simulink model "IEEE39_IBR_FrequencyControl_Fullversion_2020b"  (R2020b)
settings: Solver=VariableStepAuto  StartTime=0.0  StopTime=30  RelTol=1e-3
InitFcn:
  | IEEE39data_FrencyControl_full_Opensource;
undefined symbols (not defined in the file): alpha, c, eps_ps, eps_u, Fref, IBR_data, line, Sbase, t_start_disturbance, t_startcontrol, Vbase
libraries: powerlib x202, powerlib_meascontrol x81, powerlib_extras x27, pid_lib x14, simulink x4
(part 5 of 5)

== system IEEE39_IBR_FrequencyControl_Fullversion_2020b/G6_GFL/PV_PQ3/Subsystem2/Subsystem1 ==
  P_ref : Inport
  Q_ref : Inport  Port=2
  Ud : Inport  Port=3
  Divide5 : Product  Inputs=*/
  Divide6 : Product  Inputs=*/
  Gain1 : Gain  Gain=-2/3
  Gain2 : Gain  Gain=2/3
  Id_ref : Outport  VectorParamsAs1DForOutWhenUnconnected=off
  Iq_ref : Outport  Port=2  VectorParamsAs1DForOutWhenUnconnected=off
  wires:
  Q_ref/1 -> Divide6/1
  Divide6/1 -> Gain1/1
  P_ref/1 -> Divide5/1
  Gain1/1 -> Iq_ref/1
  Divide5/1 -> Gain2/1
  Gain2/1 -> Id_ref/1
  Ud/1 -> Divide6/2, Divide5/2

== system IEEE39_IBR_FrequencyControl_Fullversion_2020b/G6_GFL/PV_PQ3/Subsystem2/WL ==
  In1 : Inport
  freq : Inport  Port=2
  L : Inport  Port=3
  2pai : Constant  Value=2*pi
  Product : Product  Inputs=**
  Product1 : Product  Inputs=***
  Out1 : Outport  VectorParamsAs1DForOutWhenUnconnected=off
  wires:
  2pai/1 -> Product/2
  L/1 -> Product1/3
  freq/1 -> Product/1
  Product1/1 -> Out1/1
  Product/1 -> Product1/2
  In1/1 -> Product1/1

== system IEEE39_IBR_FrequencyControl_Fullversion_2020b/G6_GFL/PV_PQ3/Subsystem2/WL1 ==
  In1 : Inport
  freq : Inport  Port=2
  L : Inport  Port=3
  2pai : Constant  Value=2*pi
  Product : Product
  Product1 : Product  Inputs=3
  Out1 : Outport  VectorParamsAs1DForOutWhenUnconnected=off
  wires:
  2pai/1 -> Product/2
  L/1 -> Product1/3
  freq/1 -> Product/1
  Product1/1 -> Out1/1
  Product/1 -> Product1/2
  In1/1 -> Product1/1

== system IEEE39_IBR_FrequencyControl_Fullversion_2020b/GFM1/PV_PQ3/Freq_Droop/Subsystem1 ==
  w : Inport
  Add4 : Sum
  Clock : Clock
  Constant : Constant  Value=0
  Constant1 : Constant  Value=IBR_data(10,4)
  Constant2 : Constant  Value=IBR_data(10,5)
  Difference : simulink/Discrete/Difference  ICPrevInput=0.0  OutMin=[]  OutMax=[]  OutDataType=fixdt(1, 16)  OutScaling=2^-10  DoSatur=off
  Divide1 : Product  Inputs=**
  Divide3 : Product  Inputs=**
  Subsystem : Subsystem
  Switch : Switch  Criteria=u2 > Threshold  Threshold=t_startcontrol  ZeroCross=off
  Out1 : Outport
  tag scope: deltaP10_GFM=global
  wires:
  Subsystem/1(delatPset) -> Switch/1
  Divide1/1 -> Add4/1
  Switch/1 -> Out1/1, [deltaP10_GFM]
  Divide3/1 -> Difference/1
  Constant/1 -> Switch/3
  Add4/1 -> Subsystem/1(Dw)
  Clock/1 -> Switch/2
  Constant1/1 -> Divide1/1
  Constant2/1 -> Divide3/1
  Difference/1 -> Add4/2
  w/1 -> Subsystem/2(w), Divide3/2, Divide1/2

== system IEEE39_IBR_FrequencyControl_Fullversion_2020b/GFM1/PV_PQ3/V//F/Subsystem ==
  note: w
  eo : Inport
  io : Inport  Port=2
  i : Inport  Port=3
  f : Inport  Port=4
  Init_Phase_degree : Inport  Port=5
  Add : Sum
  Demux : Demux  Outputs=3
  Demux1 : Demux  Outputs=3
  Demux2 : Demux  Outputs=3
  Gain1 : Gain  Gain=2*pi
  Gain2 : Gain  Gain=pi/180
  Integrator : Integrator
  Terminator1 : Terminator
  Terminator2 : Terminator
  Terminator3 : Terminator
  abc to dq0 : powerlib_meascontrol/Transformations/abc to dq0  Alignment=90 degrees behind phase A axis
  abc to dq1 : powerlib_meascontrol/Transformations/abc to dq0  Alignment=90 degrees behind phase A axis
  abc to dq2 : powerlib_meascontrol/Transformations/abc to dq0  Alignment=90 degrees behind phase A axis
  eod : Outport  VectorParamsAs1DForOutWhenUnconnected=off
  eoq : Outport  Port=2  VectorParamsAs1DForOutWhenUnconnected=off
  iod : Outport  Port=3  VectorParamsAs1DForOutWhenUnconnected=off
  ioq : Outport  Port=4  VectorParamsAs1DForOutWhenUnconnected=off
  id : Outport  Port=5  VectorParamsAs1DForOutWhenUnconnected=off
  iq : Outport  Port=6  VectorParamsAs1DForOutWhenUnconnected=off
  w : Outport  Port=7  VectorParamsAs1DForOutWhenUnconnected=off
  "wt " : Outport  Port=8  VectorParamsAs1DForOutWhenUnconnected=off
  wires:
  eo/1 -> abc to dq0/1
  i/1 -> abc to dq1/1
  f/1 -> Gain1/1
  Add/1 -> "wt "/1, abc to dq1/2, abc to dq2/2, abc to dq0/2
  Demux1/1 -> id/1
  Demux1/2 -> iq/1
  Demux1/3 -> Terminator3/1
  Demux/1 -> eod/1
  Demux/2 -> eoq/1
  Demux/3 -> Terminator1/1
  io/1 -> abc to dq2/1
  Demux2/3 -> Terminator2/1
  Gain1/1 -> Integrator/1, w/1
  Demux2/1 -> iod/1
  Demux2/2 -> ioq/1
  abc to dq2/1 -> Demux2/1
  abc to dq1/1 -> Demux1/1
  abc to dq0/1 -> Demux/1
  Integrator/1 -> Add/1
  Init_Phase_degree/1 -> Gain2/1
  Gain2/1 -> Add/2

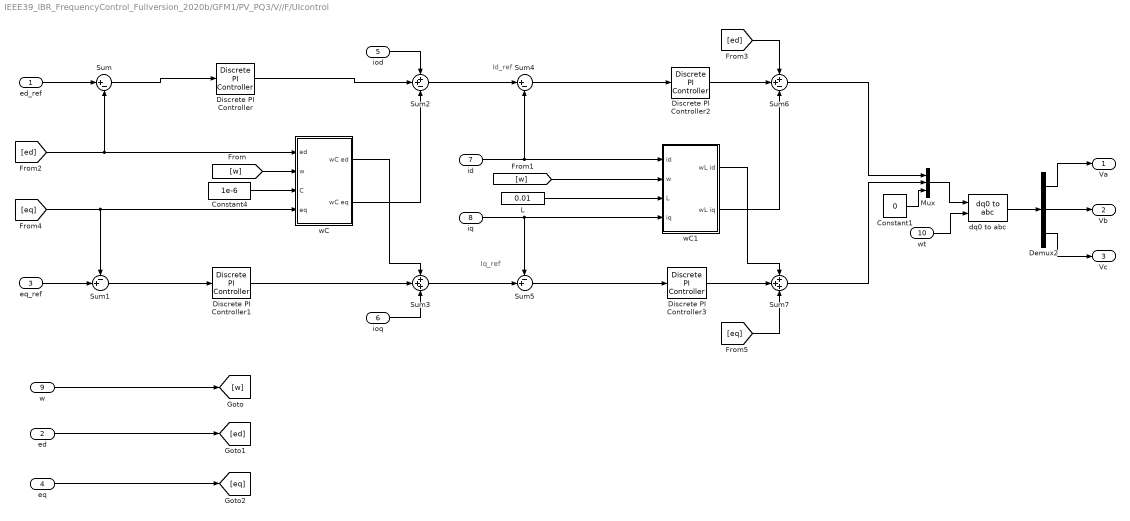
== system IEEE39_IBR_FrequencyControl_Fullversion_2020b/GFM1/PV_PQ3/V//F/UIcontrol ==
  note: Id_ref
  note: Iq_ref
  ed_ref : Inport
  ed : Inport  Port=2
  eq_ref : Inport  Port=3
  eq : Inport  Port=4
  iod : Inport  Port=5
  ioq : Inport  Port=6
  id : Inport  Port=7
  iq : Inport  Port=8
  w : Inport  Port=9
  "wt " : Inport  Port=10
  Constant1 : Constant  Value=0
  Constant4 : Constant  Value=1e-6
  Demux2 : Demux  Outputs=3
  Discrete PI Controller : powerlib_extras/Discrete  Control Blocks/Discrete PI Controller  Kp=0.3  Ki=0.8  Par_Limits=[1e6 -1e6]  Init=0  Ts=2e-4
  Discrete PI Controller1 : powerlib_extras/Discrete  Control Blocks/Discrete PI Controller  Kp=0.3  Ki=0.8  Par_Limits=[1e6 -1e6]  Init=0  Ts=2e-4
  Discrete PI Controller2 : powerlib_extras/Discrete  Control Blocks/Discrete PI Controller  Kp=2.5  Ki=12.5  Par_Limits=[1e6 -1e6]  Init=0  Ts=2e-4
  Discrete PI Controller3 : powerlib_extras/Discrete  Control Blocks/Discrete PI Controller  Kp=2.5  Ki=12.5  Par_Limits=[1e6 -1e6]  Init=0  Ts=2e-4
  L : Constant  Value=0.01
  Mux : Mux  Inputs=3
  Sum : Sum  Inputs=|+-
  Sum1 : Sum  Inputs=-+|
  Sum2 : Sum  Inputs=++-
  Sum3 : Sum  Inputs=+++
  Sum4 : Sum  Inputs=|+-
  Sum5 : Sum  Inputs=-+|
  Sum6 : Sum  Inputs=++-
  Sum7 : Sum  Inputs=+++
  dq0 to abc : powerlib_meascontrol/Transformations/dq0 to abc  Alignment=90 degrees behind phase A axis
  wC : Subsystem
  wC1 : Subsystem
  Va : Outport
  Vb : Outport  Port=2
  Vc : Outport  Port=3
  wires:
  [ed] -> wC/1(ed), Sum/2
  Mux/1 -> dq0 to abc/1
  Demux2/1 -> Va/1
  Demux2/2 -> Vb/1
  Demux2/3 -> Vc/1
  dq0 to abc/1 -> Demux2/1
  Constant4/1 -> wC/3(C)
  [w] -> wC/2(w)
  [eq] -> wC/4(eq), Sum1/1
  eq_ref/1 -> Sum1/2
  Sum2/1 -> Sum4/1
  L/1 -> wC1/3(L)
  Discrete PI Controller3/1 -> Sum7/2
  Discrete PI Controller2/1 -> Sum6/2
  w/1 -> [w]
  [w] -> wC1/2(w)
  ed/1 -> [ed]
  eq/1 -> [eq]
  Sum6/1 -> Mux/1
  Sum7/1 -> Mux/2
  Sum3/1 -> Sum5/2
  Constant1/1 -> Mux/3
  iq/1 -> Sum5/1, wC1/4(iq)
  [eq] -> Sum7/3
  [ed] -> Sum6/1
  id/1 -> wC1/1(id), Sum4/2
  wC/1(wC ed) -> Sum3/1
  ioq/1 -> Sum3/3
  iod/1 -> Sum2/1
  wC/2(wC eq) -> Sum2/3
  wC1/1(wL id) -> Sum7/1
  wC1/2(wL iq) -> Sum6/3
  Sum/1 -> Discrete PI Controller/1
  Discrete PI Controller/1 -> Sum2/2
  Sum1/1 -> Discrete PI Controller1/1
  Discrete PI Controller1/1 -> Sum3/2
  Sum4/1 -> Discrete PI Controller2/1
  Sum5/1 -> Discrete PI Controller3/1
  ed_ref/1 -> Sum/1
  "wt "/1 -> dq0 to abc/2

== system IEEE39_IBR_FrequencyControl_Fullversion_2020b/GFM2/PV_PQ3/Freq_Droop/Subsystem1 ==
  w : Inport
  Add4 : Sum
  Clock : Clock
  Constant : Constant  Value=0
  Constant1 : Constant  Value=IBR_data(9,4)
  Constant2 : Constant  Value=IBR_data(10,5)
  Difference : simulink/Discrete/Difference  ICPrevInput=0.0  OutMin=[]  OutMax=[]  OutDataType=fixdt(1, 16)  OutScaling=2^-10  DoSatur=off
  Divide1 : Product  Inputs=**
  Divide3 : Product  Inputs=**
  Subsystem : Subsystem
  Switch : Switch  Criteria=u2 > Threshold  Threshold=t_startcontrol  ZeroCross=off
  Out1 : Outport
  tag scope: deltaP9_GFM=global
  wires:
  w/1 -> Subsystem/2(w), Divide3/2, Divide1/2
  Subsystem/1(delatPset) -> Switch/1
  Divide1/1 -> Add4/1
  Switch/1 -> Out1/1, [deltaP9_GFM]
  Divide3/1 -> Difference/1
  Constant/1 -> Switch/3
  Add4/1 -> Subsystem/1(Dw)
  Clock/1 -> Switch/2
  Constant1/1 -> Divide1/1
  Constant2/1 -> Divide3/1
  Difference/1 -> Add4/2

== system IEEE39_IBR_FrequencyControl_Fullversion_2020b/GFM2/PV_PQ3/V//F/Subsystem ==
  note: w
  eo : Inport
  io : Inport  Port=2
  i : Inport  Port=3
  f : Inport  Port=4
  Init_Phase_degree : Inport  Port=5
  Add : Sum
  Demux : Demux  Outputs=3
  Demux1 : Demux  Outputs=3
  Demux2 : Demux  Outputs=3
  Gain1 : Gain  Gain=2*pi
  Gain2 : Gain  Gain=pi/180
  Integrator : Integrator
  Scope2 : Scope
  Terminator1 : Terminator
  Terminator2 : Terminator
  Terminator3 : Terminator
  abc to dq0 : powerlib_meascontrol/Transformations/abc to dq0  Alignment=90 degrees behind phase A axis
  abc to dq1 : powerlib_meascontrol/Transformations/abc to dq0  Alignment=90 degrees behind phase A axis
  abc to dq2 : powerlib_meascontrol/Transformations/abc to dq0  Alignment=90 degrees behind phase A axis
  eod : Outport  VectorParamsAs1DForOutWhenUnconnected=off
  eoq : Outport  Port=2  VectorParamsAs1DForOutWhenUnconnected=off
  iod : Outport  Port=3  VectorParamsAs1DForOutWhenUnconnected=off
  ioq : Outport  Port=4  VectorParamsAs1DForOutWhenUnconnected=off
  id : Outport  Port=5  VectorParamsAs1DForOutWhenUnconnected=off
  iq : Outport  Port=6  VectorParamsAs1DForOutWhenUnconnected=off
  w : Outport  Port=7  VectorParamsAs1DForOutWhenUnconnected=off
  "wt " : Outport  Port=8  VectorParamsAs1DForOutWhenUnconnected=off
  wires:
  eo/1 -> abc to dq0/1
  i/1 -> abc to dq1/1
  f/1 -> Gain1/1
  Add/1 -> "wt "/1, abc to dq1/2, abc to dq2/2, abc to dq0/2
  Demux1/1 -> id/1
  Demux1/2 -> iq/1
  Demux1/3 -> Terminator3/1
  Demux/1 -> eod/1
  Demux/2 -> eoq/1
  Demux/3 -> Terminator1/1
  io/1 -> abc to dq2/1
  Demux2/3 -> Terminator2/1
  Gain1/1 -> Integrator/1, w/1
  Demux2/1 -> iod/1
  Demux2/2 -> ioq/1
  abc to dq2/1 -> Demux2/1
  abc to dq1/1 -> Demux1/1
  abc to dq0/1 -> Demux/1
  Integrator/1 -> Add/1
  Init_Phase_degree/1 -> Gain2/1
  Gain2/1 -> Add/2, Scope2/1

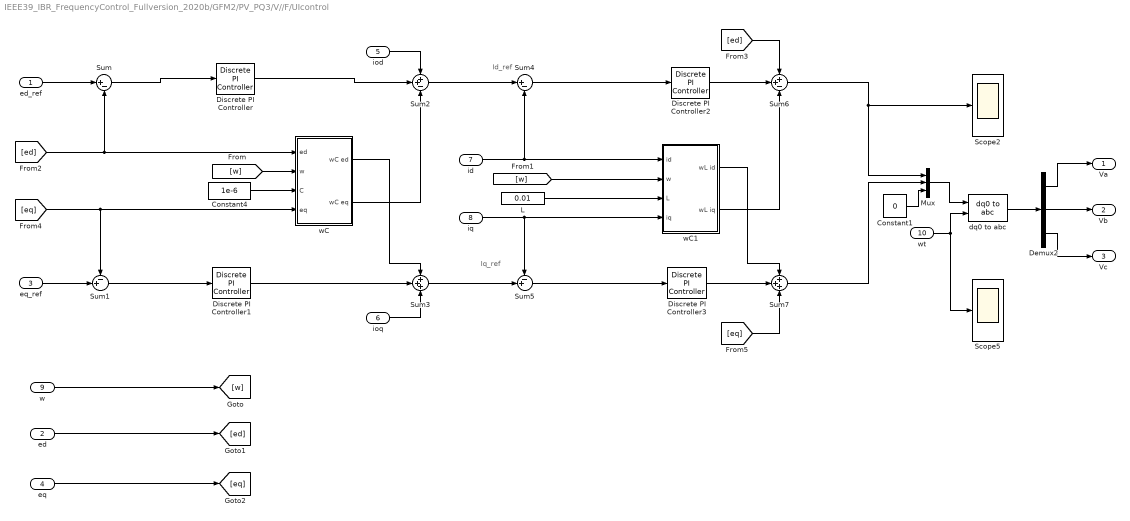
== system IEEE39_IBR_FrequencyControl_Fullversion_2020b/GFM2/PV_PQ3/V//F/UIcontrol ==
  note: Id_ref
  note: Iq_ref
  ed_ref : Inport
  ed : Inport  Port=2
  eq_ref : Inport  Port=3
  eq : Inport  Port=4
  iod : Inport  Port=5
  ioq : Inport  Port=6
  id : Inport  Port=7
  iq : Inport  Port=8
  w : Inport  Port=9
  "wt " : Inport  Port=10
  Constant1 : Constant  Value=0
  Constant4 : Constant  Value=1e-6
  Demux2 : Demux  Outputs=3
  Discrete PI Controller : powerlib_extras/Discrete  Control Blocks/Discrete PI Controller  Kp=0.3  Ki=0.8  Par_Limits=[1e6 -1e6]  Init=0  Ts=2e-4
  Discrete PI Controller1 : powerlib_extras/Discrete  Control Blocks/Discrete PI Controller  Kp=0.3  Ki=0.8  Par_Limits=[1e6 -1e6]  Init=0  Ts=2e-4
  Discrete PI Controller2 : powerlib_extras/Discrete  Control Blocks/Discrete PI Controller  Kp=2.5  Ki=12.5  Par_Limits=[1e6 -1e6]  Init=0  Ts=2e-4
  Discrete PI Controller3 : powerlib_extras/Discrete  Control Blocks/Discrete PI Controller  Kp=2.5  Ki=12.5  Par_Limits=[1e6 -1e6]  Init=0  Ts=2e-4
  L : Constant  Value=0.01
  Mux : Mux  Inputs=3
  Scope2 : Scope
  Scope5 : Scope
  Sum : Sum  Inputs=|+-
  Sum1 : Sum  Inputs=-+|
  Sum2 : Sum  Inputs=++-
  Sum3 : Sum  Inputs=+++
  Sum4 : Sum  Inputs=|+-
  Sum5 : Sum  Inputs=-+|
  Sum6 : Sum  Inputs=++-
  Sum7 : Sum  Inputs=+++
  dq0 to abc : powerlib_meascontrol/Transformations/dq0 to abc  Alignment=90 degrees behind phase A axis
  wC : Subsystem
  wC1 : Subsystem
  Va : Outport
  Vb : Outport  Port=2
  Vc : Outport  Port=3
  wires:
  [ed] -> wC/1(ed), Sum/2
  Mux/1 -> dq0 to abc/1
  Demux2/1 -> Va/1
  Demux2/2 -> Vb/1
  Demux2/3 -> Vc/1
  dq0 to abc/1 -> Demux2/1
  Constant4/1 -> wC/3(C)
  [w] -> wC/2(w)
  [eq] -> wC/4(eq), Sum1/1
  eq_ref/1 -> Sum1/2
  Sum2/1 -> Sum4/1
  L/1 -> wC1/3(L)
  Discrete PI Controller3/1 -> Sum7/2
  Discrete PI Controller2/1 -> Sum6/2
  w/1 -> [w]
  [w] -> wC1/2(w)
  ed/1 -> [ed]
  eq/1 -> [eq]
  Sum6/1 -> Scope2/1, Mux/1
  Sum7/1 -> Mux/2
  Sum3/1 -> Sum5/2
  Constant1/1 -> Mux/3
  iq/1 -> Sum5/1, wC1/4(iq)
  [eq] -> Sum7/3
  [ed] -> Sum6/1
  id/1 -> wC1/1(id), Sum4/2
  wC/1(wC ed) -> Sum3/1
  ioq/1 -> Sum3/3
  iod/1 -> Sum2/1
  wC/2(wC eq) -> Sum2/3
  wC1/1(wL id) -> Sum7/1
  wC1/2(wL iq) -> Sum6/3
  Sum/1 -> Discrete PI Controller/1
  Discrete PI Controller/1 -> Sum2/2
  Sum1/1 -> Discrete PI Controller1/1
  Discrete PI Controller1/1 -> Sum3/2
  Sum4/1 -> Discrete PI Controller2/1
  Sum5/1 -> Discrete PI Controller3/1
  ed_ref/1 -> Sum/1
  "wt "/1 -> Scope5/1, dq0 to abc/2

== system IEEE39_IBR_FrequencyControl_Fullversion_2020b/GFM3/PV_PQ3/Freq_Droop/Subsystem1 ==
  w : Inport
  Add4 : Sum
  Clock : Clock
  Constant : Constant  Value=0
  Constant1 : Constant  Value=IBR_data(8,4)
  Constant2 : Constant  Value=IBR_data(10,5)
  Difference : simulink/Discrete/Difference  ICPrevInput=0.0  OutMin=[]  OutMax=[]  OutDataType=fixdt(1, 16)  OutScaling=2^-10  DoSatur=off
  Divide1 : Product  Inputs=**
  Divide3 : Product  Inputs=**
  Subsystem : Subsystem
  Switch : Switch  Criteria=u2 > Threshold  Threshold=t_startcontrol  ZeroCross=off
  Out1 : Outport
  tag scope: deltaP8_GFM=global
  wires:
  w/1 -> Subsystem/2(w), Divide3/2, Divide1/2
  Subsystem/1(delatPset) -> Switch/1
  Divide1/1 -> Add4/1
  Switch/1 -> Out1/1, [deltaP8_GFM]
  Divide3/1 -> Difference/1
  Constant/1 -> Switch/3
  Add4/1 -> Subsystem/1(Dw)
  Clock/1 -> Switch/2
  Constant1/1 -> Divide1/1
  Constant2/1 -> Divide3/1
  Difference/1 -> Add4/2

== system IEEE39_IBR_FrequencyControl_Fullversion_2020b/GFM3/PV_PQ3/V//F/Subsystem ==
  note: w
  eo : Inport
  io : Inport  Port=2
  i : Inport  Port=3
  f : Inport  Port=4
  Init_Phase_degree : Inport  Port=5
  Add : Sum
  Demux : Demux  Outputs=3
  Demux1 : Demux  Outputs=3
  Demux2 : Demux  Outputs=3
  Gain1 : Gain  Gain=2*pi
  Gain2 : Gain  Gain=pi/180
  Integrator : Integrator
  Scope2 : Scope
  Terminator1 : Terminator
  Terminator2 : Terminator
  Terminator3 : Terminator
  abc to dq0 : powerlib_meascontrol/Transformations/abc to dq0  Alignment=90 degrees behind phase A axis
  abc to dq1 : powerlib_meascontrol/Transformations/abc to dq0  Alignment=90 degrees behind phase A axis
  abc to dq2 : powerlib_meascontrol/Transformations/abc to dq0  Alignment=90 degrees behind phase A axis
  eod : Outport  VectorParamsAs1DForOutWhenUnconnected=off
  eoq : Outport  Port=2  VectorParamsAs1DForOutWhenUnconnected=off
  iod : Outport  Port=3  VectorParamsAs1DForOutWhenUnconnected=off
  ioq : Outport  Port=4  VectorParamsAs1DForOutWhenUnconnected=off
  id : Outport  Port=5  VectorParamsAs1DForOutWhenUnconnected=off
  iq : Outport  Port=6  VectorParamsAs1DForOutWhenUnconnected=off
  w : Outport  Port=7  VectorParamsAs1DForOutWhenUnconnected=off
  "wt " : Outport  Port=8  VectorParamsAs1DForOutWhenUnconnected=off
  wires:
  eo/1 -> abc to dq0/1
  i/1 -> abc to dq1/1
  f/1 -> Gain1/1
  Add/1 -> "wt "/1, abc to dq1/2, abc to dq2/2, abc to dq0/2
  Demux1/1 -> id/1
  Demux1/2 -> iq/1
  Demux1/3 -> Terminator3/1
  Demux/1 -> eod/1
  Demux/2 -> eoq/1
  Demux/3 -> Terminator1/1
  io/1 -> abc to dq2/1
  Demux2/3 -> Terminator2/1
  Gain1/1 -> Integrator/1, w/1
  Demux2/1 -> iod/1
  Demux2/2 -> ioq/1
  abc to dq2/1 -> Demux2/1
  abc to dq1/1 -> Demux1/1
  abc to dq0/1 -> Demux/1
  Integrator/1 -> Add/1
  Init_Phase_degree/1 -> Gain2/1
  Gain2/1 -> Add/2, Scope2/1

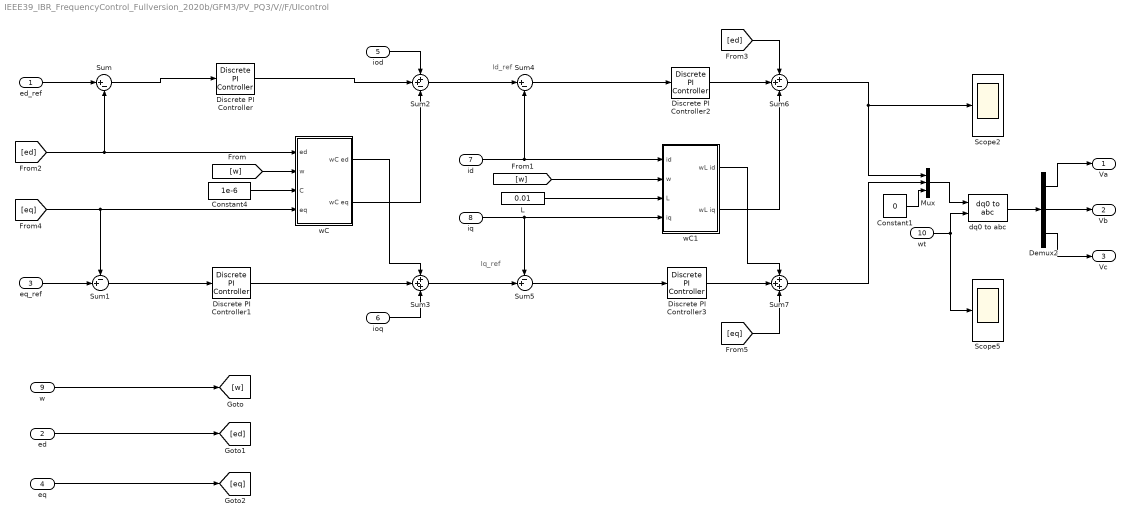
== system IEEE39_IBR_FrequencyControl_Fullversion_2020b/GFM3/PV_PQ3/V//F/UIcontrol ==
  note: Id_ref
  note: Iq_ref
  ed_ref : Inport
  ed : Inport  Port=2
  eq_ref : Inport  Port=3
  eq : Inport  Port=4
  iod : Inport  Port=5
  ioq : Inport  Port=6
  id : Inport  Port=7
  iq : Inport  Port=8
  w : Inport  Port=9
  "wt " : Inport  Port=10
  Constant1 : Constant  Value=0
  Constant4 : Constant  Value=1e-6
  Demux2 : Demux  Outputs=3
  Discrete PI Controller : powerlib_extras/Discrete  Control Blocks/Discrete PI Controller  Kp=0.3  Ki=0.8  Par_Limits=[1e6 -1e6]  Init=0  Ts=2e-4
  Discrete PI Controller1 : powerlib_extras/Discrete  Control Blocks/Discrete PI Controller  Kp=0.3  Ki=0.8  Par_Limits=[1e6 -1e6]  Init=0  Ts=2e-4
  Discrete PI Controller2 : powerlib_extras/Discrete  Control Blocks/Discrete PI Controller  Kp=2.5  Ki=12.5  Par_Limits=[1e6 -1e6]  Init=0  Ts=2e-4
  Discrete PI Controller3 : powerlib_extras/Discrete  Control Blocks/Discrete PI Controller  Kp=2.5  Ki=12.5  Par_Limits=[1e6 -1e6]  Init=0  Ts=2e-4
  L : Constant  Value=0.01
  Mux : Mux  Inputs=3
  Scope2 : Scope
  Scope5 : Scope
  Sum : Sum  Inputs=|+-
  Sum1 : Sum  Inputs=-+|
  Sum2 : Sum  Inputs=++-
  Sum3 : Sum  Inputs=+++
  Sum4 : Sum  Inputs=|+-
  Sum5 : Sum  Inputs=-+|
  Sum6 : Sum  Inputs=++-
  Sum7 : Sum  Inputs=+++
  dq0 to abc : powerlib_meascontrol/Transformations/dq0 to abc  Alignment=90 degrees behind phase A axis
  wC : Subsystem
  wC1 : Subsystem
  Va : Outport
  Vb : Outport  Port=2
  Vc : Outport  Port=3
  wires:
  [ed] -> wC/1(ed), Sum/2
  Mux/1 -> dq0 to abc/1
  Demux2/1 -> Va/1
  Demux2/2 -> Vb/1
  Demux2/3 -> Vc/1
  dq0 to abc/1 -> Demux2/1
  Constant4/1 -> wC/3(C)
  [w] -> wC/2(w)
  [eq] -> wC/4(eq), Sum1/1
  eq_ref/1 -> Sum1/2
  Sum2/1 -> Sum4/1
  L/1 -> wC1/3(L)
  Discrete PI Controller3/1 -> Sum7/2
  Discrete PI Controller2/1 -> Sum6/2
  w/1 -> [w]
  [w] -> wC1/2(w)
  ed/1 -> [ed]
  eq/1 -> [eq]
  Sum6/1 -> Scope2/1, Mux/1
  Sum7/1 -> Mux/2
  Sum3/1 -> Sum5/2
  Constant1/1 -> Mux/3
  iq/1 -> Sum5/1, wC1/4(iq)
  [eq] -> Sum7/3
  [ed] -> Sum6/1
  id/1 -> wC1/1(id), Sum4/2
  wC/1(wC ed) -> Sum3/1
  ioq/1 -> Sum3/3
  iod/1 -> Sum2/1
  wC/2(wC eq) -> Sum2/3
  wC1/1(wL id) -> Sum7/1
  wC1/2(wL iq) -> Sum6/3
  Sum/1 -> Discrete PI Controller/1
  Discrete PI Controller/1 -> Sum2/2
  Sum1/1 -> Discrete PI Controller1/1
  Discrete PI Controller1/1 -> Sum3/2
  Sum4/1 -> Discrete PI Controller2/1
  Sum5/1 -> Discrete PI Controller3/1
  ed_ref/1 -> Sum/1
  "wt "/1 -> Scope5/1, dq0 to abc/2

== system IEEE39_IBR_FrequencyControl_Fullversion_2020b/GFM4/PV_PQ3/Freq_Droop/Subsystem1 ==
  w : Inport
  Add4 : Sum
  Clock : Clock
  Constant : Constant  Value=0
  Constant1 : Constant  Value=IBR_data(7,4)
  Constant2 : Constant  Value=IBR_data(10,5)
  Difference : simulink/Discrete/Difference  ICPrevInput=0.0  OutMin=[]  OutMax=[]  OutDataType=fixdt(1, 16)  OutScaling=2^-10  DoSatur=off
  Divide1 : Product  Inputs=**
  Divide3 : Product  Inputs=**
  Subsystem : Subsystem
  Switch : Switch  Criteria=u2 > Threshold  Threshold=t_startcontrol  ZeroCross=off
  Out1 : Outport
  tag scope: deltaP7_GFM=global
  wires:
  w/1 -> Subsystem/2(w), Divide3/2, Divide1/2
  Subsystem/1(delatPset) -> Switch/1
  Divide1/1 -> Add4/1
  Switch/1 -> Out1/1, [deltaP7_GFM]
  Divide3/1 -> Difference/1
  Constant/1 -> Switch/3
  Add4/1 -> Subsystem/1(Dw)
  Clock/1 -> Switch/2
  Constant1/1 -> Divide1/1
  Constant2/1 -> Divide3/1
  Difference/1 -> Add4/2

== system IEEE39_IBR_FrequencyControl_Fullversion_2020b/GFM4/PV_PQ3/V//F/Subsystem ==
  note: w
  eo : Inport
  io : Inport  Port=2
  i : Inport  Port=3
  f : Inport  Port=4
  Init_Phase_degree : Inport  Port=5
  Add : Sum
  Demux : Demux  Outputs=3
  Demux1 : Demux  Outputs=3
  Demux2 : Demux  Outputs=3
  Gain1 : Gain  Gain=2*pi
  Gain2 : Gain  Gain=pi/180
  Integrator : Integrator
  Scope2 : Scope
  Terminator1 : Terminator
  Terminator2 : Terminator
  Terminator3 : Terminator
  abc to dq0 : powerlib_meascontrol/Transformations/abc to dq0  Alignment=90 degrees behind phase A axis
  abc to dq1 : powerlib_meascontrol/Transformations/abc to dq0  Alignment=90 degrees behind phase A axis
  abc to dq2 : powerlib_meascontrol/Transformations/abc to dq0  Alignment=90 degrees behind phase A axis
  eod : Outport  VectorParamsAs1DForOutWhenUnconnected=off
  eoq : Outport  Port=2  VectorParamsAs1DForOutWhenUnconnected=off
  iod : Outport  Port=3  VectorParamsAs1DForOutWhenUnconnected=off
  ioq : Outport  Port=4  VectorParamsAs1DForOutWhenUnconnected=off
  id : Outport  Port=5  VectorParamsAs1DForOutWhenUnconnected=off
  iq : Outport  Port=6  VectorParamsAs1DForOutWhenUnconnected=off
  w : Outport  Port=7  VectorParamsAs1DForOutWhenUnconnected=off
  "wt " : Outport  Port=8  VectorParamsAs1DForOutWhenUnconnected=off
  wires:
  eo/1 -> abc to dq0/1
  i/1 -> abc to dq1/1
  f/1 -> Gain1/1
  Add/1 -> "wt "/1, abc to dq1/2, abc to dq2/2, abc to dq0/2
  Demux1/1 -> id/1
  Demux1/2 -> iq/1
  Demux1/3 -> Terminator3/1
  Demux/1 -> eod/1
  Demux/2 -> eoq/1
  Demux/3 -> Terminator1/1
  io/1 -> abc to dq2/1
  Demux2/3 -> Terminator2/1
  Gain1/1 -> Integrator/1, w/1
  Demux2/1 -> iod/1
  Demux2/2 -> ioq/1
  abc to dq2/1 -> Demux2/1
  abc to dq1/1 -> Demux1/1
  abc to dq0/1 -> Demux/1
  Integrator/1 -> Add/1
  Init_Phase_degree/1 -> Gain2/1
  Gain2/1 -> Add/2, Scope2/1

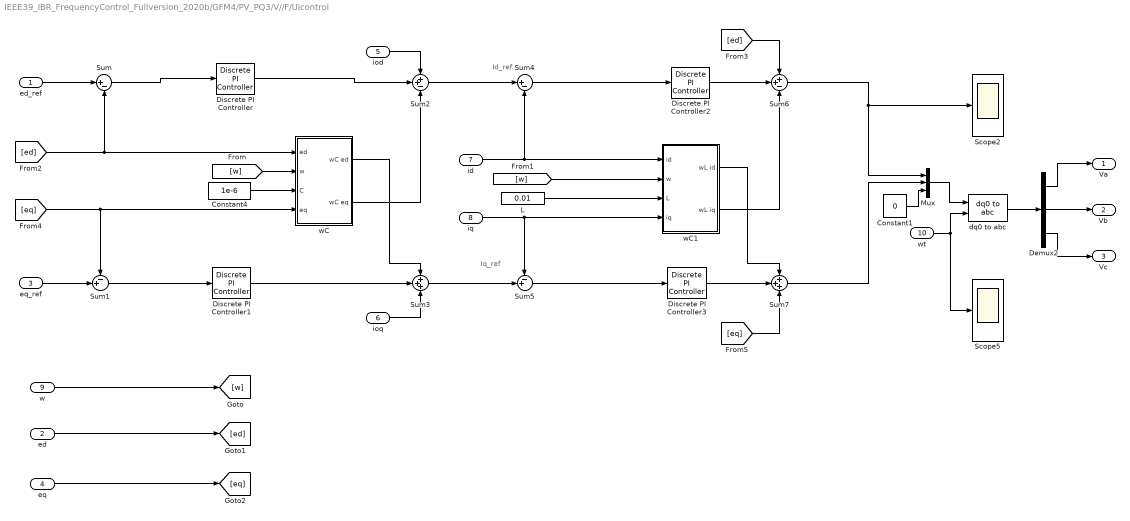
== system IEEE39_IBR_FrequencyControl_Fullversion_2020b/GFM4/PV_PQ3/V//F/UIcontrol ==
  note: Id_ref
  note: Iq_ref
  ed_ref : Inport
  ed : Inport  Port=2
  eq_ref : Inport  Port=3
  eq : Inport  Port=4
  iod : Inport  Port=5
  ioq : Inport  Port=6
  id : Inport  Port=7
  iq : Inport  Port=8
  w : Inport  Port=9
  "wt " : Inport  Port=10
  Constant1 : Constant  Value=0
  Constant4 : Constant  Value=1e-6
  Demux2 : Demux  Outputs=3
  Discrete PI Controller : powerlib_extras/Discrete  Control Blocks/Discrete PI Controller  Kp=0.3  Ki=0.8  Par_Limits=[1e6 -1e6]  Init=0  Ts=2e-4
  Discrete PI Controller1 : powerlib_extras/Discrete  Control Blocks/Discrete PI Controller  Kp=0.3  Ki=0.8  Par_Limits=[1e6 -1e6]  Init=0  Ts=2e-4
  Discrete PI Controller2 : powerlib_extras/Discrete  Control Blocks/Discrete PI Controller  Kp=2.5  Ki=12.5  Par_Limits=[1e6 -1e6]  Init=0  Ts=2e-4
  Discrete PI Controller3 : powerlib_extras/Discrete  Control Blocks/Discrete PI Controller  Kp=2.5  Ki=12.5  Par_Limits=[1e6 -1e6]  Init=0  Ts=2e-4
  L : Constant  Value=0.01
  Mux : Mux  Inputs=3
  Scope2 : Scope
  Scope5 : Scope
  Sum : Sum  Inputs=|+-
  Sum1 : Sum  Inputs=-+|
  Sum2 : Sum  Inputs=++-
  Sum3 : Sum  Inputs=+++
  Sum4 : Sum  Inputs=|+-
  Sum5 : Sum  Inputs=-+|
  Sum6 : Sum  Inputs=++-
  Sum7 : Sum  Inputs=+++
  dq0 to abc : powerlib_meascontrol/Transformations/dq0 to abc  Alignment=90 degrees behind phase A axis
  wC : Subsystem
  wC1 : Subsystem
  Va : Outport
  Vb : Outport  Port=2
  Vc : Outport  Port=3
  wires:
  [ed] -> wC/1(ed), Sum/2
  Mux/1 -> dq0 to abc/1
  Demux2/1 -> Va/1
  Demux2/2 -> Vb/1
  Demux2/3 -> Vc/1
  dq0 to abc/1 -> Demux2/1
  Constant4/1 -> wC/3(C)
  [w] -> wC/2(w)
  [eq] -> wC/4(eq), Sum1/1
  eq_ref/1 -> Sum1/2
  Sum2/1 -> Sum4/1
  L/1 -> wC1/3(L)
  Discrete PI Controller3/1 -> Sum7/2
  Discrete PI Controller2/1 -> Sum6/2
  w/1 -> [w]
  [w] -> wC1/2(w)
  ed/1 -> [ed]
  eq/1 -> [eq]
  Sum6/1 -> Scope2/1, Mux/1
  Sum7/1 -> Mux/2
  Sum3/1 -> Sum5/2
  Constant1/1 -> Mux/3
  iq/1 -> Sum5/1, wC1/4(iq)
  [eq] -> Sum7/3
  [ed] -> Sum6/1
  id/1 -> wC1/1(id), Sum4/2
  wC/1(wC ed) -> Sum3/1
  ioq/1 -> Sum3/3
  iod/1 -> Sum2/1
  wC/2(wC eq) -> Sum2/3
  wC1/1(wL id) -> Sum7/1
  wC1/2(wL iq) -> Sum6/3
  Sum/1 -> Discrete PI Controller/1
  Discrete PI Controller/1 -> Sum2/2
  Sum1/1 -> Discrete PI Controller1/1
  Discrete PI Controller1/1 -> Sum3/2
  Sum4/1 -> Discrete PI Controller2/1
  Sum5/1 -> Discrete PI Controller3/1
  ed_ref/1 -> Sum/1
  "wt "/1 -> Scope5/1, dq0 to abc/2

== system IEEE39_IBR_FrequencyControl_Fullversion_2020b/PV/PV_PQ3/Subsystem2/Subsystem1 ==
  P_ref : Inport
  Q_ref : Inport  Port=2
  Ud : Inport  Port=3
  Divide5 : Product  Inputs=*/
  Divide6 : Product  Inputs=*/
  Gain1 : Gain  Gain=-2/3
  Gain2 : Gain  Gain=2/3
  Id_ref : Outport  VectorParamsAs1DForOutWhenUnconnected=off
  Iq_ref : Outport  Port=2  VectorParamsAs1DForOutWhenUnconnected=off
  wires:
  Q_ref/1 -> Divide6/1
  Divide6/1 -> Gain1/1
  P_ref/1 -> Divide5/1
  Gain1/1 -> Iq_ref/1
  Divide5/1 -> Gain2/1
  Gain2/1 -> Id_ref/1
  Ud/1 -> Divide6/2, Divide5/2

== system IEEE39_IBR_FrequencyControl_Fullversion_2020b/PV/PV_PQ3/Subsystem2/WL ==
  In1 : Inport
  freq : Inport  Port=2
  L : Inport  Port=3
  2pai : Constant  Value=2*pi
  Product : Product  Inputs=**
  Product1 : Product  Inputs=***
  Out1 : Outport  VectorParamsAs1DForOutWhenUnconnected=off
  wires:
  2pai/1 -> Product/2
  L/1 -> Product1/3
  freq/1 -> Product/1
  Product1/1 -> Out1/1
  Product/1 -> Product1/2
  In1/1 -> Product1/1

== system IEEE39_IBR_FrequencyControl_Fullversion_2020b/PV/PV_PQ3/Subsystem2/WL1 ==
  In1 : Inport
  freq : Inport  Port=2
  L : Inport  Port=3
  2pai : Constant  Value=2*pi
  Product : Product
  Product1 : Product  Inputs=3
  Out1 : Outport  VectorParamsAs1DForOutWhenUnconnected=off
  wires:
  2pai/1 -> Product/2
  L/1 -> Product1/3
  freq/1 -> Product/1
  Product1/1 -> Out1/1
  Product/1 -> Product1/2
  In1/1 -> Product1/1

== system IEEE39_IBR_FrequencyControl_Fullversion_2020b/GFM1/PV_PQ3/Freq_Droop/Subsystem1/Subsystem ==
  Dw : Inport
  w : Inport  Port=2
  Add1 : Sum
  Add2 : Sum  Inputs=+++
  Add3 : Sum  Inputs=-+
  Gain : Gain  Gain=eps_u
  Gain1 : Gain  Gain=eps_ps
  Gain2 : Gain  Gain=c(10)
  Gain3 : Gain  Gain=alpha
  Integrator : Integrator  ExternalReset=rising  ZeroCross=off
  Integrator1 : Integrator  ExternalReset=rising  ZeroCross=off
  Saturation : Saturate  UpperLimit=IBR_data(10,6)-IBR_data(10,10)  LowerLimit=IBR_data(10,6)-IBR_data(10,9)
  Step : Step  Time=3  SampleTime=0
  Step1 : Step  Time=3  SampleTime=0
  delatPset : Outport
  wires:
  w/1 -> Add2/3
  Gain2/1 -> Add2/1
  Integrator1/1 -> delatPset/1, Add3/1, Add1/1, Gain2/1
  Step/1 -> Integrator1/2
  Step1/1 -> Integrator/2
  Integrator/1 -> Gain/1
  Gain/1 -> Add2/2
  Dw/1 -> Integrator/1
  Gain1/1 -> Integrator1/1
  Add2/1 -> Gain3/1
  Gain3/1 -> Add1/2
  Add1/1 -> Saturation/1
  Saturation/1 -> Add3/2
  Add3/1 -> Gain1/1

== system IEEE39_IBR_FrequencyControl_Fullversion_2020b/GFM1/PV_PQ3/V//F/UIcontrol/wC ==
  ed : Inport
  w : Inport  Port=2
  C : Inport  Port=3
  eq : Inport  Port=4
  Product1 : Product  Inputs=3
  Product2 : Product  Inputs=3
  wC ed : Outport  VectorParamsAs1DForOutWhenUnconnected=off
  wC eq : Outport  Port=2  VectorParamsAs1DForOutWhenUnconnected=off
  wires:
  C/1 -> Product1/3, Product2/2
  Product1/1 -> wC ed/1
  w/1 -> Product1/2, Product2/1
  ed/1 -> Product1/1
  eq/1 -> Product2/3
  Product2/1 -> wC eq/1

== system IEEE39_IBR_FrequencyControl_Fullversion_2020b/GFM1/PV_PQ3/V//F/UIcontrol/wC1 ==
  id : Inport
  w : Inport  Port=2
  L : Inport  Port=3
  iq : Inport  Port=4
  Product1 : Product  Inputs=***
  Product2 : Product  Inputs=***
  wL id : Outport  VectorParamsAs1DForOutWhenUnconnected=off
  wL iq : Outport  Port=2  VectorParamsAs1DForOutWhenUnconnected=off
  wires:
  L/1 -> Product1/3, Product2/2
  Product1/1 -> wL id/1
  w/1 -> Product1/2, Product2/1
  id/1 -> Product1/1
  iq/1 -> Product2/3
  Product2/1 -> wL iq/1

== system IEEE39_IBR_FrequencyControl_Fullversion_2020b/GFM2/PV_PQ3/Freq_Droop/Subsystem1/Subsystem ==
  Dw : Inport
  w : Inport  Port=2
  Add1 : Sum
  Add2 : Sum  Inputs=+++
  Add3 : Sum  Inputs=-+
  Gain : Gain  Gain=eps_u
  Gain1 : Gain  Gain=eps_ps
  Gain2 : Gain  Gain=c(9)
  Gain3 : Gain  Gain=alpha
  Integrator : Integrator  ExternalReset=rising  ZeroCross=off
  Integrator1 : Integrator  ExternalReset=rising  ZeroCross=off
  Saturation : Saturate  UpperLimit=IBR_data(9,6)-IBR_data(9,10)  LowerLimit=IBR_data(9,6)-IBR_data(9,9)
  Step : Step  Time=3  SampleTime=0
  Step1 : Step  Time=3  SampleTime=0
  delatPset : Outport
  wires:
  w/1 -> Add2/3
  Gain2/1 -> Add2/1
  Integrator1/1 -> delatPset/1, Add3/1, Add1/1, Gain2/1
  Step/1 -> Integrator1/2
  Step1/1 -> Integrator/2
  Integrator/1 -> Gain/1
  Gain/1 -> Add2/2
  Dw/1 -> Integrator/1
  Gain1/1 -> Integrator1/1
  Add2/1 -> Gain3/1
  Gain3/1 -> Add1/2
  Add1/1 -> Saturation/1
  Saturation/1 -> Add3/2
  Add3/1 -> Gain1/1

== system IEEE39_IBR_FrequencyControl_Fullversion_2020b/GFM2/PV_PQ3/V//F/UIcontrol/wC ==
  ed : Inport
  w : Inport  Port=2
  C : Inport  Port=3
  eq : Inport  Port=4
  Product1 : Product  Inputs=3
  Product2 : Product  Inputs=3
  wC ed : Outport  VectorParamsAs1DForOutWhenUnconnected=off
  wC eq : Outport  Port=2  VectorParamsAs1DForOutWhenUnconnected=off
  wires:
  C/1 -> Product1/3, Product2/2
  Product1/1 -> wC ed/1
  w/1 -> Product1/2, Product2/1
  ed/1 -> Product1/1
  eq/1 -> Product2/3
  Product2/1 -> wC eq/1

== system IEEE39_IBR_FrequencyControl_Fullversion_2020b/GFM2/PV_PQ3/V//F/UIcontrol/wC1 ==
  id : Inport
  w : Inport  Port=2
  L : Inport  Port=3
  iq : Inport  Port=4
  Product1 : Product  Inputs=***
  Product2 : Product  Inputs=***
  wL id : Outport  VectorParamsAs1DForOutWhenUnconnected=off
  wL iq : Outport  Port=2  VectorParamsAs1DForOutWhenUnconnected=off
  wires:
  L/1 -> Product1/3, Product2/2
  Product1/1 -> wL id/1
  w/1 -> Product1/2, Product2/1
  id/1 -> Product1/1
  iq/1 -> Product2/3
  Product2/1 -> wL iq/1

== system IEEE39_IBR_FrequencyControl_Fullversion_2020b/GFM3/PV_PQ3/Freq_Droop/Subsystem1/Subsystem ==
  Dw : Inport
  w : Inport  Port=2
  Add1 : Sum
  Add2 : Sum  Inputs=+++
  Add3 : Sum  Inputs=-+
  Gain : Gain  Gain=eps_u
  Gain1 : Gain  Gain=eps_ps
  Gain2 : Gain  Gain=c(8)
  Gain3 : Gain  Gain=alpha
  Integrator : Integrator  ExternalReset=rising  ZeroCross=off
  Integrator1 : Integrator  ExternalReset=rising  ZeroCross=off
  Saturation : Saturate  UpperLimit=IBR_data(8,6)-IBR_data(8,10)  LowerLimit=IBR_data(8,6)-IBR_data(8,9)
  Step : Step  Time=3  SampleTime=0
  Step1 : Step  Time=3  SampleTime=0
  delatPset : Outport
  wires:
  w/1 -> Add2/3
  Gain2/1 -> Add2/1
  Integrator1/1 -> delatPset/1, Add3/1, Add1/1, Gain2/1
  Step/1 -> Integrator1/2
  Step1/1 -> Integrator/2
  Integrator/1 -> Gain/1
  Gain/1 -> Add2/2
  Dw/1 -> Integrator/1
  Gain1/1 -> Integrator1/1
  Add2/1 -> Gain3/1
  Gain3/1 -> Add1/2
  Add1/1 -> Saturation/1
  Saturation/1 -> Add3/2
  Add3/1 -> Gain1/1

== system IEEE39_IBR_FrequencyControl_Fullversion_2020b/GFM3/PV_PQ3/V//F/UIcontrol/wC ==
  ed : Inport
  w : Inport  Port=2
  C : Inport  Port=3
  eq : Inport  Port=4
  Product1 : Product  Inputs=3
  Product2 : Product  Inputs=3
  wC ed : Outport  VectorParamsAs1DForOutWhenUnconnected=off
  wC eq : Outport  Port=2  VectorParamsAs1DForOutWhenUnconnected=off
  wires:
  C/1 -> Product1/3, Product2/2
  Product1/1 -> wC ed/1
  w/1 -> Product1/2, Product2/1
  ed/1 -> Product1/1
  eq/1 -> Product2/3
  Product2/1 -> wC eq/1

== system IEEE39_IBR_FrequencyControl_Fullversion_2020b/GFM3/PV_PQ3/V//F/UIcontrol/wC1 ==
  id : Inport
  w : Inport  Port=2
  L : Inport  Port=3
  iq : Inport  Port=4
  Product1 : Product  Inputs=***
  Product2 : Product  Inputs=***
  wL id : Outport  VectorParamsAs1DForOutWhenUnconnected=off
  wL iq : Outport  Port=2  VectorParamsAs1DForOutWhenUnconnected=off
  wires:
  L/1 -> Product1/3, Product2/2
  Product1/1 -> wL id/1
  w/1 -> Product1/2, Product2/1
  id/1 -> Product1/1
  iq/1 -> Product2/3
  Product2/1 -> wL iq/1

== system IEEE39_IBR_FrequencyControl_Fullversion_2020b/GFM4/PV_PQ3/Freq_Droop/Subsystem1/Subsystem ==
  Dw : Inport
  w : Inport  Port=2
  Add1 : Sum
  Add2 : Sum  Inputs=+++
  Add3 : Sum  Inputs=-+
  Gain : Gain  Gain=eps_u
  Gain1 : Gain  Gain=eps_ps
  Gain2 : Gain  Gain=c(7)
  Gain3 : Gain  Gain=alpha
  Integrator : Integrator  ExternalReset=rising  ZeroCross=off
  Integrator1 : Integrator  ExternalReset=rising  ZeroCross=off
  Saturation : Saturate  UpperLimit=IBR_data(7,6)-IBR_data(7,10)  LowerLimit=IBR_data(7,6)-IBR_data(7,9)
  Step : Step  Time=3  SampleTime=0
  Step1 : Step  Time=3  SampleTime=0
  delatPset : Outport
  wires:
  w/1 -> Add2/3
  Gain2/1 -> Add2/1
  Integrator1/1 -> delatPset/1, Add3/1, Add1/1, Gain2/1
  Step/1 -> Integrator1/2
  Step1/1 -> Integrator/2
  Integrator/1 -> Gain/1
  Gain/1 -> Add2/2
  Dw/1 -> Integrator/1
  Gain1/1 -> Integrator1/1
  Add2/1 -> Gain3/1
  Gain3/1 -> Add1/2
  Add1/1 -> Saturation/1
  Saturation/1 -> Add3/2
  Add3/1 -> Gain1/1

== system IEEE39_IBR_FrequencyControl_Fullversion_2020b/GFM4/PV_PQ3/V//F/UIcontrol/wC ==
  ed : Inport
  w : Inport  Port=2
  C : Inport  Port=3
  eq : Inport  Port=4
  Product1 : Product  Inputs=3
  Product2 : Product  Inputs=3
  wC ed : Outport  VectorParamsAs1DForOutWhenUnconnected=off
  wC eq : Outport  Port=2  VectorParamsAs1DForOutWhenUnconnected=off
  wires:
  C/1 -> Product1/3, Product2/2
  Product1/1 -> wC ed/1
  w/1 -> Product1/2, Product2/1
  ed/1 -> Product1/1
  eq/1 -> Product2/3
  Product2/1 -> wC eq/1

== system IEEE39_IBR_FrequencyControl_Fullversion_2020b/GFM4/PV_PQ3/V//F/UIcontrol/wC1 ==
  id : Inport
  w : Inport  Port=2
  L : Inport  Port=3
  iq : Inport  Port=4
  Product1 : Product  Inputs=***
  Product2 : Product  Inputs=***
  wL id : Outport  VectorParamsAs1DForOutWhenUnconnected=off
  wL iq : Outport  Port=2  VectorParamsAs1DForOutWhenUnconnected=off
  wires:
  L/1 -> Product1/3, Product2/2
  Product1/1 -> wL id/1
  w/1 -> Product1/2, Product2/1
  id/1 -> Product1/1
  iq/1 -> Product2/3
  Product2/1 -> wL iq/1
